simulink model "Longitudinaldynamicmodel_SmartFortwo"  (R2018b)
settings: Solver=FixedStepAuto  StartTime=0.0  StopTime=1  FixedStep=0.01  RelTol=1e-3
values from neighbouring files (symbols this model uses):
  VehMass = 988.5    [Longitudinaldynamicmodel_SmartFortwo_Parameterfile.m]
undefined symbols (not defined in the file or in its folder): DiscIntNeverNeededParam
libraries: Constant_Environment x1, Driver_PI x1, Longitudinal_DrivingCycles x1, Acceleration_Calculation x1, Air_Resistance x1, Roll_Resistance x1, Slope_Resistance x1, Constant_Power_Source x1, Simple_Auxiliary x1, Electric_Drive_Tabled_Consumption x1, Gear_Stage x1, DCAC_Converter x1
(part 1 of 3)
settings Model: NumberOfSteps=1000  Creator=Tony  LastModifiedBy=ga69qig
settings SFSimCC: SimUseLocalCustomCode=off
settings RTWCC: RTWUseLocalCustomCode=off
settings CodeAppCC: StateflowObjectComments=on

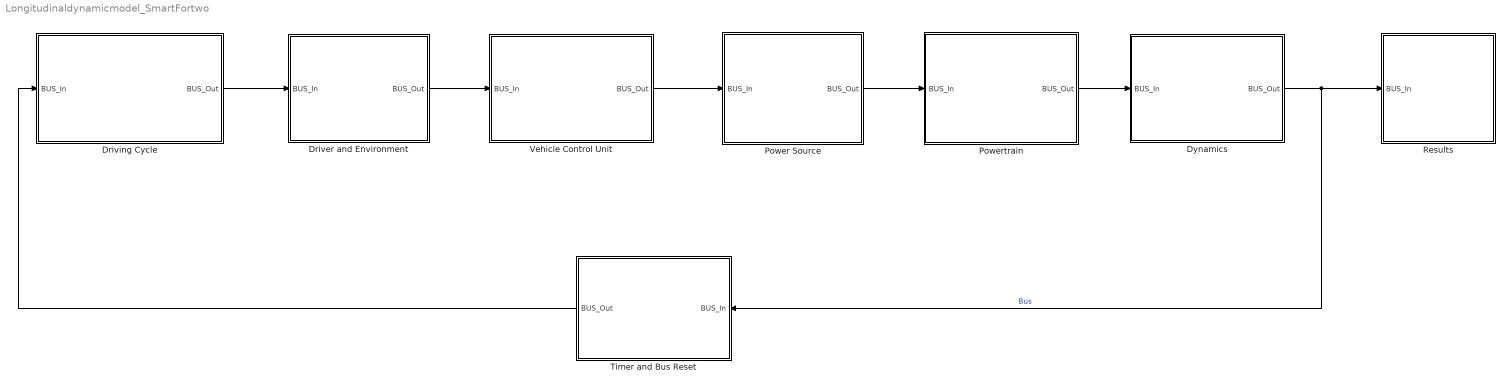
== system Longitudinaldynamicmodel_SmartFortwo ==
  Driver and Environment : Subsystem
      mask help:
      | <Author> Alexander Koch based on Stefan Müller, Stephan Rohr
      | <Date> 03/04/2017
      |
      | <Description>
      | Consist of a Bus In and a Bus Out Block. To Select Signals from the Bus open the Bus In Block, to write signals to the Bus under a certain tab name open the bus out block. For further information, please read the discription of the Bus In and Bus out Block
      |
      | The Block automaticlly disconnects the link to the library block after opening the first time
      |
      | <Parameters>
      | -
      |
      | <Inputs>
      | BUS_In [Bus]
      |
      | <Outputs>
      | Bus_Out [Bus]
      settings: OpenFcn=|
      | set_param(gcb(),'LinkStatus','none')
      | open_system(gcb(),'force')
      mask Display:
      | [picturexpos,pictureypos,picturewidth,pictureheight] = ...
      |     CalcBlockPicturePosition(gcb,1,0.01,0.1,30,30); % calculating picture position depending on Block size and minimum margin size
      | image('Driver_PI.svg',[picturexpos pictureypos picturewidth pictureheight]); % plot picture to block
  Driving Cycle : Subsystem
      mask help:
      | <Author> Alexander Koch based on Stefan Müller, Stephan Rohr
      | <Date> 03/04/2017
      |
      | <Description>
      | Consist of a Bus In and a Bus Out Block. To Select Signals from the Bus open the Bus In Block, to write signals to the Bus under a certain tab name open the bus out block. For further information, please read the discription of the Bus In and Bus out Block
      |
      | The Block automaticlly disconnects the link to the library block after opening the first time
      |
      | <Parameters>
      | -
      |
      | <Inputs>
      | BUS_In [Bus]
      |
      | <Outputs>
      | Bus_Out [Bus]
      settings: OpenFcn=|
      | set_param(gcb(),'LinkStatus','none')
      | open_system(gcb(),'force')
      mask Display:
      | [picturexpos,pictureypos,picturewidth,pictureheight] = ...
      |     CalcBlockPicturePosition(gcb,1,0.01,0.1,50,50); % calculating picture position depending on Block size and minimum margin size
      | image('Longitudinal_DrivingCycles.svg',[picturexpos pictureypos picturewidth pictureheight]); % plot picture to block
  Dynamics : Subsystem
      mask help:
      | <Author> Alexander Koch based on Stefan Müller, Stephan Rohr
      | <Date> 03/04/2017
      |
      | <Description>
      | Consist of a Bus In and a Bus Out Block. To Select Signals from the Bus open the Bus In Block, to write signals to the Bus under a certain tab name open the bus out block. For further information, please read the discription of the Bus In and Bus out Block
      |
      | The Block automaticlly disconnects the link to the library block after opening the first time
      |
      | <Parameters>
      | -
      |
      | <Inputs>
      | BUS_In [Bus]
      |
      | <Outputs>
      | Bus_Out [Bus]
      settings: OpenFcn=|
      | set_param(gcb(),'LinkStatus','none')
      | open_system(gcb(),'force')
      mask Display:
      | [picturexpos,pictureypos,picturewidth,pictureheight] = ...
      |     CalcBlockPicturePosition(gcb,1,0.01,0.1,40,50); % calculating picture position depending on Block size and minimum margin size
      | image('Acceleration_Calculation.svg',[picturexpos pictureypos picturewidth pictureheight]); % plot picture to block
  Power Source : Subsystem
      mask help:
      | <Author> Alexander Koch based on Stefan Müller, Stephan Rohr
      | <Date> 03/04/2017
      |
      | <Description>
      | Consist of a Bus In and a Bus Out Block. To Select Signals from the Bus open the Bus In Block, to write signals to the Bus under a certain tab name open the bus out block. For further information, please read the discription of the Bus In and Bus out Block
      |
      | The Block automaticlly disconnects the link to the library block after opening the first time
      |
      | <Parameters>
      | -
      |
      | <Inputs>
      | BUS_In [Bus]
      |
      | <Outputs>
      | Bus_Out [Bus]
      settings: OpenFcn=|
      | set_param(gcb(),'LinkStatus','none')
      | open_system(gcb(),'force')
      mask Display:
      | [picturexpos,pictureypos,picturewidth,pictureheight] = ...
      |     CalcBlockPicturePosition(gcb,3/6,0.01,0.1,40,40); % calculating picture position depending on Block size and minimum margin size
      | image('Constant_Power_Source.svg',[picturexpos pictureypos picturewidth pictureheight]); % plot picture to block
  Powertrain : Subsystem
      mask help:
      | <Author> Alexander Koch based on Stefan Müller, Stephan Rohr
      | <Date> 03/04/2017
      |
      | <Description>
      | Consist of a Bus In and a Bus Out Block. To Select Signals from the Bus open the Bus In Block, to write signals to the Bus under a certain tab name open the bus out block. For further information, please read the discription of the Bus In and Bus out Block
      |
      | The Block automaticlly disconnects the link to the library block after opening the first time
      |
      | <Parameters>
      | -
      |
      | <Inputs>
      | BUS_In [Bus]
      |
      | <Outputs>
      | Bus_Out [Bus]
      settings: OpenFcn=|
      | set_param(gcb(),'LinkStatus','none')
      | open_system(gcb(),'force')
      mask Display:
      | [picturexpos,pictureypos,picturewidth,pictureheight] = ...
      |     CalcBlockPicturePosition(gcb,1,0.01,0.1,40,40); % calculating picture position depending on Block size and minimum margin size
      | image('Electric_Drive_Simple_Efficiency.svg',[picturexpos pictureypos picturewidth pictureheight]); % plot picture to block
  Results : Subsystem
      mask help:
      | <Author> Alexander Koch
      | <Date> 03/04/2017
      | <Predecessor> Stefan Müller, Stephan Rohr
      |
      | <Description>
      | Consist of a Bus In and a Bus Out Block. To Select Signals from the Bus open the Bus In Block, to write signals to the Bus under a certain tab name open the bus out block. For further information, please read the discription of the Bus In and Bus out Block
      |
      | The Block automaticlly disconnects the link to the library block after opening the first time
      |
      | <Parameters>
      | -
      |
      | <Inputs>
      | Bus [Bus]
      |
      | <Outputs>
      | Bus [Bus]
      settings: OpenFcn=|
      | set_param(gcb(),'LinkStatus','none')
      | open_system(gcb(),'force')
      mask Display:
      | [picturexpos,pictureypos,picturewidth,pictureheight] = ...
      |     CalcBlockPicturePosition(gcb,1,0.01,0.1,40,10); % calculating picture position depending on Block size and minimum margin size
      | image('Scopes_Simulation.svg',[picturexpos pictureypos picturewidth pictureheight]); % plot picture to block
  Timer and Bus Reset : Subsystem
      settings: OpenFcn=|
      | set_param(gcb(),'LinkStatus','none')
      | open_system(gcb(),'mask')
      mask DialogControl RefreshBus Prompt: Refresh Bus
      mask DialogControl RefreshBus Callback: TimerandBusResetRefreshBus()
      mask Display:
      | [picturexpos,pictureypos,picturewidth,pictureheight] = ...
      |     CalcBlockPicturePosition(gcb,1,0.01,0.1,50,50); % calculating picture position depending on Block size and minimum margin size
      | image('reset.png',[picturexpos pictureypos picturewidth pictureheight]); % plot picture to block
  Vehicle Control Unit : Subsystem
      mask help:
      | <Author> Alexander Koch based on Stefan Müller, Stephan Rohr
      | <Date> 03/04/2017
      |
      | <Description>
      | Consist of a Bus In and a Bus Out Block. To Select Signals from the Bus open the Bus In Block, to write signals to the Bus under a certain tab name open the bus out block. For further information, please read the discription of the Bus In and Bus out Block
      |
      | The Block automaticlly disconnects the link to the library block after opening the first time
      |
      | <Parameters>
      | -
      |
      | <Inputs>
      | BUS_In [Bus]
      |
      | <Outputs>
      | Bus_Out [Bus]
      settings: OpenFcn=|
      | set_param(gcb(),'LinkStatus','none')
      | open_system(gcb(),'force')
      mask Display:
      | [picturexpos,pictureypos,picturewidth,pictureheight] = ...
      |     CalcBlockPicturePosition(gcb,1,0.01,0.1,30,30); % calculating picture position depending on Block size and minimum margin size
      | image('Control_Unit_Simple.svg',[picturexpos pictureypos picturewidth pictureheight]); % plot picture to block
  wires:
  Timer and Bus Reset/1(BUS_Out) -> Driving Cycle/1(BUS_In)
  Driving Cycle/1(BUS_Out) -> Driver and Environment/1(BUS_In)
  Driver and Environment/1(BUS_Out) -> Vehicle Control Unit/1(BUS_In)
  Vehicle Control Unit/1(BUS_Out) -> Power Source/1(BUS_In)
  Power Source/1(BUS_Out) -> Powertrain/1(BUS_In)
  Powertrain/1(BUS_Out) -> Dynamics/1(BUS_In)
  Dynamics/1(BUS_Out) -> Timer and Bus Reset/1(BUS_In), Results/1(BUS_In)  "Bus"

== system Longitudinaldynamicmodel_SmartFortwo/Driver and Environment ==
  BUS_In : Inport
  BUS IN : Subsystem
      mask help:
      | <Author> Alexander Koch based on Stefan Müller, Stephan Rohr
      | <Date> 02/05/2017
      |
      | <Description>
      | Automated BUS IN Block for the Bus System. After the Bus In is connected and receives signals it is possible to choose the required signals by clicking on the block. After choosing the signals it is possible to push the Refresh button. This button builds the required amount of outputs, connects the Bus Selector and the Outputs and rename all the outputs with the corresponding signal name.
      |
      | The Block automaticlly disconnects the link to the library block after opening the first time
      |
      | <Parameters>
      | -
      |
      | <Inputs>
      | Bus [Bus]
      |
      | <Outputs>
      | Bus [Bus]
      | SignalName[-]
      mask init:
      | BusInInitFct()
      settings: OpenFcn=|
      | set_param(gcb(),'LinkStatus','none')
      | open_system(gcb(),'mask')
      | open_system(strcat(gcb(),'/Bus Selector'),'Parameter')
      mask DialogControl ParameterGroupVar Prompt: Refresh
      mask DialogControl RefreshOutputs Prompt: Refresh all Output Names
      mask DialogControl RefreshOutputs Callback: BusInInitFct()
  BUS OUT : Subsystem  mask{NumberofInputs=6, NameSys='Driver and Enironment'}
      mask prompts: NumberofInputs "Numper of costum inputs"; NameSys "Name of Bus Subsystem"
      mask help:
      | <Author> Alexander Koch based on Stefan Müller, Stephan Rohr
      | <Date> 02/05/2017
      |
      | <Description>
      | Automated BUS Out Block for the Bus System. Allows to enter the Number of costum inputs and the name of the bus system. After entering the parameters the required amout of Inputs are built and connected to the Bus Creator. The signal names that are connected to the inputs In1, ..., InN are automatically adopted at the Bus signal names and can be found in the Bus under the name of the Bus Subsystem. If the signal (line) to the Inport has no name, the name of the previous blocks outport is taken. If this is not possible, the name if the previous block is taken for the Bus signal name.
      |
      | Additional, there are two buttons. The Refresh Input Names refreshes all Input Names. This is required if signal names are changed or signals are connected for the first time. To build a new system or if another Subsystem is added between existing subsystems, the Refresh Bus Selector is required at every subsystem that is calculated after the new subsystem.
      |
      | The Block automaticlly disconnects the link to the library block after opening the first time
      |
      | <Parameters>
      | Number of costum inputs [-]
      | Name of Bus Subsystem ['abc']
      |
      | <Inputs>
      | Bus [Bus]
      | In1 [ ]
      |
      | <Outputs>
      | Bus [Bus]
      mask init:
      | BusRefreshInputs()
      settings: OpenFcn=|
      | set_param(gcb(),'LinkStatus','none')
      | open_system(gcb(),'mask')
      mask DialogControl Container3 Prompt: Refresh
      mask DialogControl RefreshInputNames Prompt: Refresh Input Names
      mask DialogControl RefreshInputNames Callback: BusRefreshLineNames()
      mask DialogControl RefreshBusSelector Prompt: Refresh Bus Selector
      mask DialogControl RefreshBusSelector Callback: BusRefreshBusSelector()
  Constant Environment : Constant_Environment/Constant Environment  Ground_Slope=0  Long_Wind_Speed=0  Ambient_P=101325  Ambient_Temp=293.15  LocalSampleTime=-1
  Driver PI : Driver_PI/Driver PI  ThrottleP=7  ThrottleI=1  BrakeP=7  BrakeI=1.5  WeightingFactorPrecontrol=0  MaxVehicleSpeed=80  hysteresis=0.05  LocalSampleTime=-1
  BUS_Out : Outport
  wires:
  BUS IN/1(BUS) -> BUS OUT/1(BUS)
  BUS OUT/1(BUS_OUT) -> BUS_Out/1
  BUS_In/1 -> BUS IN/1(BUS_In)
  BUS IN/2(v [m/s]) -> Driver PI/1
  Driver PI/1 -> BUS OUT/2(In1)
  Driver PI/2 -> BUS OUT/3(In2)
  Constant Environment/1 -> BUS OUT/4(In3)
  Constant Environment/2 -> BUS OUT/5(In4)
  BUS IN/3(VehSpd [m/s]) -> Driver PI/2
  Constant Environment/3 -> BUS OUT/6(In5)
  Constant Environment/4 -> BUS OUT/7(In6)

== system Longitudinaldynamicmodel_SmartFortwo/Driving Cycle ==
  BUS_In : Inport
  BUS IN : Subsystem
      mask help:
      | <Author> Alexander Koch
      | <Date> 02/05/2017
      | <Predecessor> Stefan Müller, Stephan Rohr
      |
      | <Description>
      | Automated BUS IN Block for the Bus System. After the Bus In is connected and receives signals it is possible to choose the required signals by clicking on the block. After choosing the signals it is possible to push the Refresh button. This button builds the required amount of outputs, connects the Bus Selector and the Outputs and rename all the outputs with the corresponding signal name.
      |
      | The Block automaticlly disconnects the link to the library block after opening the first time
      |
      | <Parameters>
      | -
      |
      | <Inputs>
      | Bus [Bus]
      |
      | <Outputs>
      | Bus [Bus]
      | SignalName[-]
      mask init:
      | BusInInitFct()
      settings: OpenFcn=|
      | set_param(gcb(),'LinkStatus','none')
      | open_system(gcb(),'mask')
      | open_system(strcat(gcb(),'/Bus Selector'),'Parameter')
      mask DialogControl ParameterGroupVar Prompt: Refresh
      mask DialogControl RefreshOutputs Prompt: Refresh all Output Names
      mask DialogControl RefreshOutputs Callback: BusInInitFct()
  BUS OUT : Subsystem  mask{NumberofInputs=4, NameSys='DrivinCycle'}
      mask prompts: NumberofInputs "Numper of costum inputs"; NameSys "Name of Bus Subsystem"
      mask help:
      | <Author> Alexander Koch based on Stefan Müller, Stephan Rohr
      | <Date> 02/05/2017
      |
      | <Description>
      | Automated BUS Out Block for the Bus System. Allows to enter the Number of costum inputs and the name of the bus system. After entering the parameters the required amout of Inputs are built and connected to the Bus Creator. The signal names that are connected to the inputs In1, ..., InN are automatically adopted at the Bus signal names and can be found in the Bus under the name of the Bus Subsystem. If the signal (line) to the Inport has no name, the name of the previous blocks outport is taken. If this is not possible, the name if the previous block is taken for the Bus signal name.
      |
      | Additional, there are two buttons. The Refresh Input Names refreshes all Input Names. This is required if signal names are changed or signals are connected for the first time. To build a new system or if another Subsystem is added between existing subsystems, the Refresh Bus Selector is required at every subsystem that is calculated after the new subsystem.
      |
      | The Block automaticlly disconnects the link to the library block after opening the first time
      |
      | <Parameters>
      | Number of costum inputs [-]
      | Name of Bus Subsystem ['abc']
      |
      | <Inputs>
      | Bus [Bus]
      | In1 [ ]
      |
      | <Outputs>
      | Bus [Bus]
      mask init:
      | BusRefreshInputs()
      settings: OpenFcn=|
      | set_param(gcb(),'LinkStatus','none')
      | open_system(gcb(),'mask')
      mask DialogControl Container3 Prompt: Refresh
      mask DialogControl RefreshInputNames Prompt: Refresh Input Names
      mask DialogControl RefreshInputNames Callback: BusRefreshLineNames()
      mask DialogControl RefreshBusSelector Prompt: Refresh Bus Selector
      mask DialogControl RefreshBusSelector Callback: BusRefreshBusSelector()
  Longitudinal Driving Cycles : Longitudinal_DrivingCycles/Longitudinal Driving Cycles  dcname=Custom_Driving_Cycle  dccircuits=1  dc_speed=cycle  dc_gear=[]  LocalSampleTime=-1
  Terminator : Terminator
  BUS_Out : Outport
  wires:
  BUS IN/1(BUS) -> BUS OUT/1(BUS)
  BUS OUT/1(BUS_OUT) -> BUS_Out/1
  BUS_In/1 -> BUS IN/1(BUS_In)
  Longitudinal Driving Cycles/1 -> BUS OUT/2(In1)  "v [m/s]"
  Longitudinal Driving Cycles/2 -> BUS OUT/3(In2)
  Longitudinal Driving Cycles/3 -> BUS OUT/4(In3)
  Longitudinal Driving Cycles/4 -> BUS OUT/5(In4)
  BUS IN/2(VehSpd [m/s]) -> Terminator/1

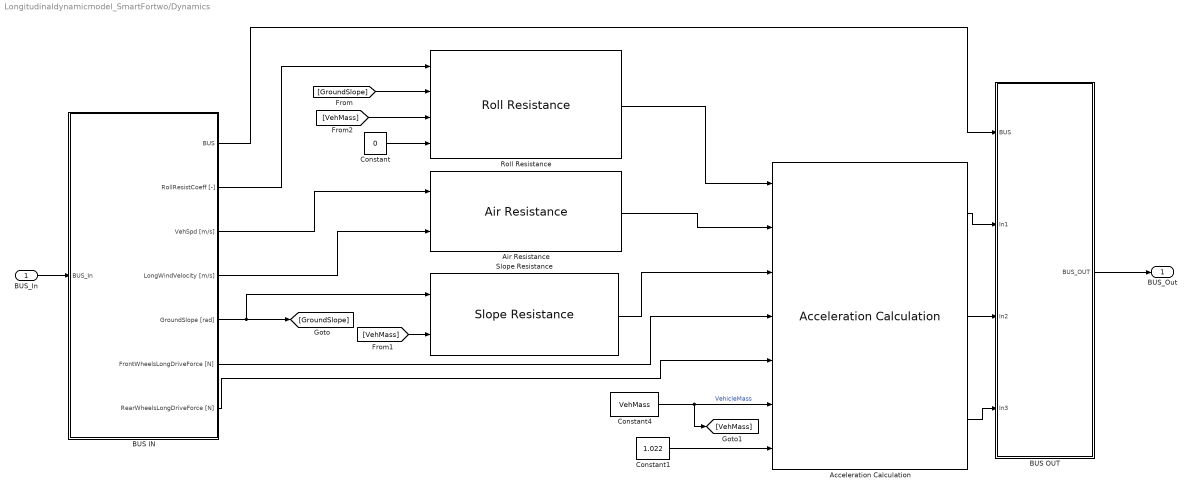
== system Longitudinaldynamicmodel_SmartFortwo/Dynamics ==
  BUS_In : Inport
  Acceleration Calculation : Acceleration_Calculation/Acceleration Calculation  InitialCondition=0  LocalSampleTime=-1
  Air Resistance : Air_Resistance/Air Resistance  A_st=1.947  Roh_Air=rho_L  c_w=0.37  LocalSampleTime=-1
  BUS IN : Subsystem
      mask help:
      | <Author> Alexander Koch
      | <Date> 02/05/2017
      | <Predecessor> Stefan Müller, Stephan Rohr
      |
      | <Description>
      | Automated BUS IN Block for the Bus System. After the Bus In is connected and receives signals it is possible to choose the required signals by clicking on the block. After choosing the signals it is possible to push the Refresh button. This button builds the required amount of outputs, connects the Bus Selector and the Outputs and rename all the outputs with the corresponding signal name.
      |
      | The Block automaticlly disconnects the link to the library block after opening the first time
      |
      | <Parameters>
      | -
      |
      | <Inputs>
      | Bus [Bus]
      |
      | <Outputs>
      | Bus [Bus]
      | SignalName[-]
      mask init:
      | BusInInitFct()
      settings: OpenFcn=|
      | set_param(gcb(),'LinkStatus','none')
      | open_system(gcb(),'mask')
      | open_system(strcat(gcb(),'/Bus Selector'),'Parameter')
      mask DialogControl ParameterGroupVar Prompt: Refresh
      mask DialogControl RefreshOutputs Prompt: Refresh all Output Names
      mask DialogControl RefreshOutputs Callback: BusInInitFct()
  BUS OUT : Subsystem  mask{NumberofInputs=3, NameSys='Dynamics'}
      mask prompts: NumberofInputs "Numper of costum inputs"; NameSys "Name of Bus Subsystem"
      mask help:
      | <Author> Alexander Koch
      | <Date> 02/05/2017
      | <Predecessor> Stefan Müller, Stephan Rohr
      |
      | <Description>
      | Automated BUS Out Block for the Bus System. Allows to enter the Number of costum inputs and the name of the bus system. After entering the parameters the required amout of Inputs are built and connected to the Bus Creator. The signal names that are connected to the inputs In1, ..., InN are automatically adopted at the Bus signal names and can be found in the Bus under the name of the Bus Subsystem. If the signal (line) to the Inport has no name, the name of the previous blocks outport is taken. If this is not possible, the name if the previous block is taken for the Bus signal name.
      |
      | Additional, there are two buttons. The Refresh Input Names refreshes all Input Names. This is required if signal names are changed or signals are connected for the first time. To build a new system or if another Subsystem is added between existing subsystems, the Refresh Bus Selector is required at every subsystem that is calculated after the new subsystem.
      |
      | The Block automaticlly disconnects the link to the library block after opening the first time
      |
      | <Parameters>
      | Number of costum inputs [-]
      | Name of Bus Subsystem ['abc']
      |
      | <Inputs>
      | Bus [Bus]
      | In1 [ ]
      |
      | <Outputs>
      | Bus [Bus]
      mask init:
      | BusRefreshInputs()
      settings: OpenFcn=|
      | set_param(gcb(),'LinkStatus','none')
      | open_system(gcb(),'mask')
      mask DialogControl Container3 Prompt: Refresh
      mask DialogControl RefreshInputNames Prompt: Refresh Input Names
      mask DialogControl RefreshInputNames Callback: BusRefreshLineNames()
      mask DialogControl RefreshBusSelector Prompt: Refresh Bus Selector
      mask DialogControl RefreshBusSelector Callback: BusRefreshBusSelector()
  Constant : Constant  Value=0
  Constant1 : Constant  Value=1.022
  Constant4 : Constant  Value=VehMass  SampleTime=-1
  Roll Resistance : Roll_Resistance/Roll Resistance  Gravity=gravity  LocalSampleTime=-1
  Slope Resistance : Slope_Resistance/Slope Resistance  Gravity=gravity  LocalSampleTime=-1
  BUS_Out : Outport
  wires:
  BUS IN/1(BUS) -> BUS OUT/1(BUS)
  BUS OUT/1(BUS_OUT) -> BUS_Out/1
  BUS_In/1 -> BUS IN/1(BUS_In)
  BUS IN/2(RollResistCoeff [-]) -> Roll Resistance/1
  Roll Resistance/1 -> Acceleration Calculation/1
  BUS IN/4(LongWindVelocity [m/s]) -> Air Resistance/2
  [GroundSlope] -> Roll Resistance/2
  BUS IN/5(GroundSlope [rad]) -> Slope Resistance/1, [GroundSlope]
  Air Resistance/1 -> Acceleration Calculation/2
  Slope Resistance/1 -> Acceleration Calculation/3
  BUS IN/6(FrontWheelsLongDriveForce [N]) -> Acceleration Calculation/4
  BUS IN/7(RearWheelsLongDriveForce [N]) -> Acceleration Calculation/5
  Constant4/1 -> [VehMass], Acceleration Calculation/6  "VehicleMass"
  [VehMass] -> Slope Resistance/2
  [VehMass] -> Roll Resistance/3
  Constant/1 -> Roll Resistance/4
  Constant1/1 -> Acceleration Calculation/7
  Acceleration Calculation/1 -> BUS OUT/2(In1)
  Acceleration Calculation/2 -> BUS OUT/3(In2)
  Acceleration Calculation/3 -> BUS OUT/4(In3)
  BUS IN/3(VehSpd [m/s]) -> Air Resistance/1

== system Longitudinaldynamicmodel_SmartFortwo/Power Source ==
  note: During the experiments the vehicle Smart Fortwo
      | was pluged in to a battery simulator, which provides
      | a power source with constant voltage.
  BUS_In : Inport
  Add : Sum
  BUS IN : Subsystem
      mask help:
      | <Author> Alexander Koch based on Stefan Müller, Stephan Rohr
      | <Date> 02/05/2017
      |
      | <Description>
      | Automated BUS IN Block for the Bus System. After the Bus In is connected and receives signals it is possible to choose the required signals by clicking on the block. After choosing the signals it is possible to push the Refresh button. This button builds the required amount of outputs, connects the Bus Selector and the Outputs and rename all the outputs with the corresponding signal name.
      |
      | The Block automaticlly disconnects the link to the library block after opening the first time
      |
      | <Parameters>
      | -
      |
      | <Inputs>
      | Bus [Bus]
      |
      | <Outputs>
      | Bus [Bus]
      | SignalName[-]
      mask init:
      | BusInInitFct()
      settings: OpenFcn=|
      | set_param(gcb(),'LinkStatus','none')
      | open_system(gcb(),'mask')
      | open_system(strcat(gcb(),'/Bus Selector'),'Parameter')
      mask DialogControl ParameterGroupVar Prompt: Refresh
      mask DialogControl RefreshOutputs Prompt: Refresh all Output Names
      mask DialogControl RefreshOutputs Callback: BusInInitFct()
  BUS OUT : Subsystem  mask{NumberofInputs=3, NameSys='Powersource'}
      mask prompts: NumberofInputs "Numper of costum inputs"; NameSys "Name of Bus Subsystem"
      mask help:
      | <Author> Alexander Koch based on Stefan Müller, Stephan Rohr
      | <Date> 02/05/2017
      |
      | <Description>
      | Automated BUS Out Block for the Bus System. Allows to enter the Number of costum inputs and the name of the bus system. After entering the parameters the required amout of Inputs are built and connected to the Bus Creator. The signal names that are connected to the inputs In1, ..., InN are automatically adopted at the Bus signal names and can be found in the Bus under the name of the Bus Subsystem. If the signal (line) to the Inport has no name, the name of the previous blocks outport is taken. If this is not possible, the name if the previous block is taken for the Bus signal name.
      |
      | Additional, there are two buttons. The Refresh Input Names refreshes all Input Names. This is required if signal names are changed or signals are connected for the first time. To build a new system or if another Subsystem is added between existing subsystems, the Refresh Bus Selector is required at every subsystem that is calculated after the new subsystem.
      |
      | The Block automaticlly disconnects the link to the library block after opening the first time
      |
      | <Parameters>
      | Number of costum inputs [-]
      | Name of Bus Subsystem ['abc']
      |
      | <Inputs>
      | Bus [Bus]
      | In1 [ ]
      |
      | <Outputs>
      | Bus [Bus]
      mask init:
      | BusRefreshInputs()
      settings: OpenFcn=|
      | set_param(gcb(),'LinkStatus','none')
      | open_system(gcb(),'mask')
      mask DialogControl Container3 Prompt: Refresh
      mask DialogControl RefreshInputNames Prompt: Refresh Input Names
      mask DialogControl RefreshInputNames Callback: BusRefreshLineNames()
      mask DialogControl RefreshBusSelector Prompt: Refresh Bus Selector
      mask DialogControl RefreshBusSelector Callback: BusRefreshBusSelector()
  Constant Power Source : Constant_Power_Source/Constant Power Source  MaxPower=400000  MinPower=-10000  LocalSampleTime=-1
  Simple Auxiliary : Simple_Auxiliary/Simple Auxiliary  AuxPower=142.6  LocalSampleTime=-1
  BUS_Out : Outport
  wires:
  BUS IN/1(BUS) -> BUS OUT/1(BUS)
  BUS OUT/1(BUS_OUT) -> BUS_Out/1
  BUS_In/1 -> BUS IN/1(BUS_In)
  Constant Power Source/1 -> BUS OUT/2(In1)
  Constant Power Source/2 -> BUS OUT/3(In2)
  Constant Power Source/3 -> BUS OUT/4(In3)
  BUS IN/2(PowertrainPowerReq [W]) -> Add/2
  Add/1 -> Constant Power Source/1
  Simple Auxiliary/1 -> Add/1  "AuxiliariesPower [W]"
